simulink model "s_0"  (R2022a)
settings: Solver=VariableStepAuto  StartTime=0.0  StopTime=10  RelTol=1e-3
settings Model: Creator=wei  LastModifiedBy=wei

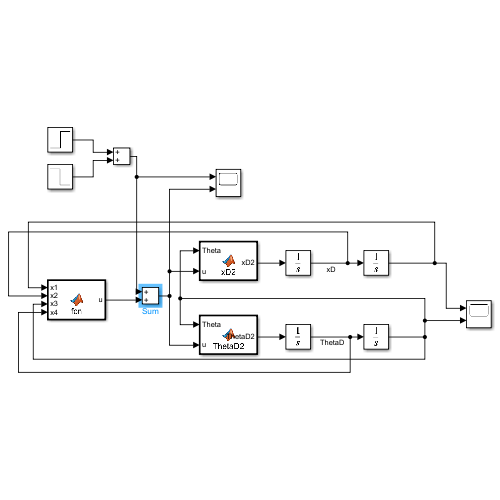
[thumbnail: Simulink's stored preview of the top-level diagram]
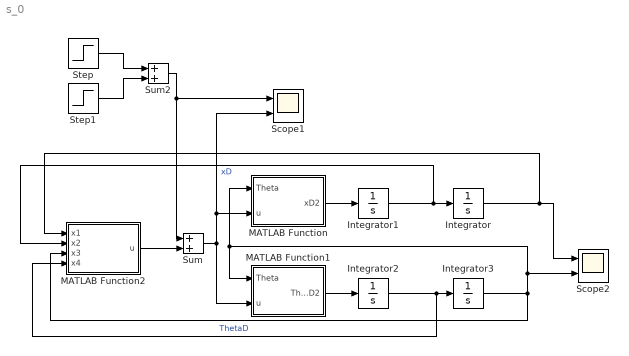
== system s_0 ==
  Integrator : Integrator
  Integrator1 : Integrator  InitialCondition=0.2
  Integrator2 : Integrator
  Integrator3 : Integrator  InitialCondition=0.2
  MATLAB Function : MATLAB Function  TreatAsAtomicUnit=on
  MATLAB Function1 : MATLAB Function  TreatAsAtomicUnit=on
  MATLAB Function2 : MATLAB Function  TreatAsAtomicUnit=on
  Scope1 : Scope  NumInputPorts=2
  Scope2 : Scope  NumInputPorts=2
  Step : Step  After=200  SampleTime=2
  Step1 : Step  After=-200  SampleTime=4
  Sum : Sum
  Sum2 : Sum
  wires:
  MATLAB Function/1(xD2) -> Integrator1/1
  Integrator3/1 -> MATLAB Function2/3(x3), Scope2/2, MATLAB Function1/1(Theta), MATLAB Function/1(Theta)
  MATLAB Function1/1(ThetaD2) -> Integrator2/1
  Integrator2/1 -> MATLAB Function2/4(x4), Integrator3/1  "ThetaD"
  Integrator1/1 -> MATLAB Function2/2(x2), Integrator/1  "xD"
  Integrator/1 -> MATLAB Function2/1(x1), Scope2/1
  Step/1 -> Sum2/1
  Sum2/1 -> Sum/1, Scope1/1
  Step1/1 -> Sum2/2
  Sum/1 -> Scope1/2, MATLAB Function/2(u), MATLAB Function1/2(u)
  MATLAB Function2/1(u) -> Sum/2

== matlab function s_0/MATLAB Function1 ==
  data: Theta input; u input; ThetaD2 output
function ThetaD2 = ThetaD2(Theta,u)

ThetaD2 = 17.97*Theta - 0.83*u;

== matlab function s_0/MATLAB Function ==
  data: Theta input; u input; xD2 output
function xD2 = xD2(Theta,u)

xD2 = -0.98*Theta + 0.5*u;

== matlab function s_0/MATLAB Function2 ==
  data: x1 input; u output; x2 input; x3 input; x4 input
function u = fcn(x1, x2, x3, x4)

K = [-487 -227 -944 -187];
X = [x1; x2; x3; x4];

u = -(K(1)*x1 + K(2)*x2 + K(3)*x3 + K(4)*x4);
